simulink subsystem "PieroControladoZ"  (R2023b)
settings: Solver=VariableStepAuto  StartTime=0.0  StopTime=10.0  RelTol=1e-3
undefined symbols (not defined in the file): DiscIntNeverNeededParam
settings Model: Creator=marqu  LastModifiedBy=marqu

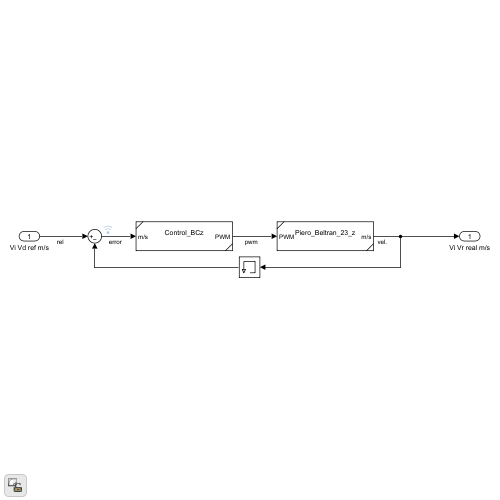
[thumbnail: Simulink's stored preview of the top-level diagram]
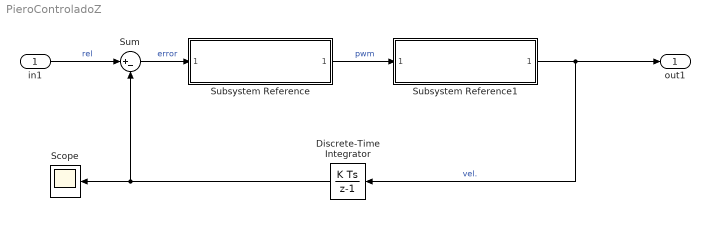
== system PieroControladoZ ==
  in1 : Inport
  Discrete-Time Integrator : DiscreteIntegrator  SampleTime=-1  ICPrevOutput=DiscIntNeverNeededParam  ICPrevScaledInput=DiscIntNeverNeededParam
  Scope : Scope
  Subsystem Reference : Subsystem  ReferencedSubsystem=Control_BCz
  Subsystem Reference1 : Subsystem  ReferencedSubsystem=Piero_Beltran_23_z
  Sum : Sum  Inputs=|+-
  out1 : Outport
  wires:
  in1/1 -> Sum/1  "rel"
  Sum/1 -> Subsystem Reference/1  "error"
  Subsystem Reference/1 -> Subsystem Reference1/1  "pwm"
  Subsystem Reference1/1 -> out1/1, Discrete-Time Integrator/1  "vel."
  Discrete-Time Integrator/1 -> Scope/1, Sum/2
